simulink model "fusionAlg"  (R2018b)
settings: Solver=FixedStepDiscrete  StartTime=0.0  StopTime=inf  FixedStep=0.01  RelTol=1e-3
PostLoadFcn:
  | if any(exist('dsrtsu_mdlpostloadfcn', 'file') ~= 0), dsrtsu_mdlpostloadfcn('Execute', bdroot); end
model workspace (MAT data in the model file):
  handle : class17 (value not decoded)
(part 8 of 24)

== system fusionAlg/FUSION /FUS_DataAdapter/VisionAdapter/ObjAdapter/Obj_39 ==
  EyeQ4_Obj_01 : Inport
  Bus Creator1 : BusCreator  Inputs=21  OutDataTypeStr=Bus: FUS_VISION_OBJ_ST
      settings: InheritFromInputs=off
  Bus Selector : BusSelector  OutputSignals=OBJ_ID,OBJ_Measuring_Status,OBJ_Object_Age,OBJ_Object_Class,OBJ_Class_Probability,OBJ_Lat_Distance,OBJ_Lat_Distance_STD,OBJ_Long_Distance,OBJ_Long_Distance_STD,OBJ_Abs_Long_Velocity,OBJ_Abs_Long_Velocity_STD,OBJ_Abs_Lat_Velocity,OBJ_Abs_Lat_Velocity_STD,OBJ_Angle_Mid,OBJ_Angle_Mid_STD,OBJ_Inv_TTC,OBJ_Inv_TTC_STD,OBJ_Abs_Long_Acc,OBJ_Abs_Long_Acc_STD,OBJ_Abs_Lat_Acc,OBJ_Abs_Lat_Acc_STD,OBJ_Length,OBJ_Width,OBJ_Height,OBJ_Heading
  Constant : Constant  OutDataTypeStr=single
  Constant1 : Constant  Value=0  OutDataTypeStr=uint8
  Constant2 : Constant  OutDataTypeStr=single
  Constant3 : Constant  Value=0  OutDataTypeStr=single
  Constant4 : Constant  Value=0  OutDataTypeStr=single
  Data Type Conversion : DataTypeConversion  OutDataTypeStr=uint32
  Data Type Conversion3 : DataTypeConversion  OutDataTypeStr=uint32
  Obj_01_Agge : Subsystem
  Obj_01_boundarhy : Subsystem
  Subsystem : Subsystem
  Subsystem1 : Subsystem
  Subsystem2 : Subsystem
  Subsystem3 : Subsystem
  Subsystem4 : Subsystem
  Subsystem5 : Subsystem
  Subsystem6 : Subsystem
  Subsystem7 : Subsystem
  Subsystem8 : Subsystem
  Obj_01_st : Outport  OutDataTypeStr=Bus: FUS_VISION_OBJ_ST
  wires:
  Bus Selector/1 -> Data Type Conversion/1  "<OBJ_ID>"
  Bus Selector/3 -> Obj_01_Agge/1(<OBJ_Object_Age>)  "<OBJ_Object_Age>"
  Obj_01_Agge/1(Obj_01_Age) -> Bus Creator1/3  "Obj_Age"
  Obj_01_boundarhy/1(Obj_01_boundary) -> Bus Creator1/4  "Obj_Boundary"
  Bus Selector/5 -> Data Type Conversion3/1  "<OBJ_Class_Probability>"
  Bus Selector/6 -> Subsystem/1(<OBJ_Lat_Distance>)  "<OBJ_Lat_Distance>"
  Bus Selector/7 -> Subsystem/2(<OBJ_Lat_Distance_STD>)  "<OBJ_Lat_Distance_STD>"
  Bus Selector/8 -> Subsystem/3(<OBJ_Long_Distance>)  "<OBJ_Long_Distance>"
  Bus Selector/9 -> Subsystem/4(<OBJ_Long_Distance_STD>)  "<OBJ_Long_Distance_STD>"
  Subsystem/1(Obj_01_coordinate) -> Bus Creator1/7  "Obj_Coor"
  Bus Selector/10 -> Subsystem1/1(<OBJ_Abs_Long_Velocity>)  "<OBJ_Abs_Long_Velocity>"
  Bus Selector/11 -> Subsystem1/2(<OBJ_Abs_Long_Velocity_STD>)  "<OBJ_Abs_Long_Velocity_STD>"
  Bus Selector/12 -> Subsystem1/3(<OBJ_Abs_Lat_Velocity>)  "<OBJ_Abs_Lat_Velocity>"
  Bus Selector/13 -> Subsystem1/4(<OBJ_Abs_Lat_Velocity_STD>)  "<OBJ_Abs_Lat_Velocity_STD>"
  Subsystem1/1(Out1) -> Bus Creator1/8  "Obj_Vel"
  Bus Selector/14 -> Subsystem2/1(<OBJ_Angle_Mid>)  "<OBJ_Angle_Mid>"
  Bus Selector/15 -> Subsystem2/2(<OBJ_Angle_Mid_STD>)  "<OBJ_Angle_Mid_STD>"
  Subsystem2/1(Out1) -> Bus Creator1/9  "Obj_Anage"
  Bus Selector/16 -> Bus Creator1/10  "<OBJ_Inv_TTC>"
  Bus Selector/17 -> Bus Creator1/11  "<OBJ_Inv_TTC_STD>"
  Bus Selector/18 -> Subsystem3/1(<OBJ_Abs_Long_Acc>)  "<OBJ_Abs_Long_Acc>"
  Bus Selector/19 -> Subsystem3/2(<OBJ_Abs_Long_Acc_STD>)  "<OBJ_Abs_Long_Acc_STD>"
  Bus Selector/20 -> Subsystem3/3(<OBJ_Abs_Lat_Acc>)  "<OBJ_Abs_Lat_Acc>"
  Bus Selector/21 -> Subsystem3/4(<OBJ_Abs_Lat_Acc_STD>)  "<OBJ_Abs_Lat_Acc_STD>"
  Subsystem3/1(Out1) -> Bus Creator1/12  "Obj_Acc"
  Constant/1 -> Bus Creator1/13  "existProb"
  Bus Selector/22 -> Subsystem4/1(<OBJ_Length>)  "<OBJ_Length>"
  Bus Selector/23 -> Subsystem4/2(<OBJ_Width>)  "<OBJ_Width>"
  Bus Selector/24 -> Subsystem4/3(<OBJ_Height>)  "<OBJ_Height>"
  Subsystem4/1(Out1) -> Bus Creator1/14  "Obj_BoxSize"
  Constant1/1 -> Bus Creator1/15  "AngelOfObj"
  Subsystem5/1(reserved1) -> Bus Creator1/16
  Bus Selector/25 -> Bus Creator1/17  "<OBJ_Heading>"
  Constant2/1 -> Bus Creator1/18
  Constant3/1 -> Bus Creator1/19
  Constant4/1 -> Bus Creator1/20
  Subsystem6/1(reserved2) -> Bus Creator1/21
  EyeQ4_Obj_01/1 -> Bus Selector/1
  Bus Creator1/1 -> Obj_01_st/1
  Data Type Conversion/1 -> Bus Creator1/1
  Data Type Conversion3/1 -> Bus Creator1/6  "Obj_TypeConf"
  Bus Selector/2 -> Subsystem7/1(<OBJ_Measuring_Status>)  "<OBJ_Measuring_Status>"
  Subsystem7/1(Obj_Status) -> Bus Creator1/2  "Obj_Status"
  Bus Selector/4 -> Subsystem8/1(<OBJ_Object_Class>)  "<OBJ_Object_Class>"
  Subsystem8/1(Obj_Type) -> Bus Creator1/5  "Obj_Type"

== system fusionAlg/FUSION /FUS_DataAdapter/VisionAdapter/ObjAdapter/Obj_4 ==
  EyeQ4_Obj_01 : Inport
  Bus Creator1 : BusCreator  Inputs=21  OutDataTypeStr=Bus: FUS_VISION_OBJ_ST
      settings: InheritFromInputs=off
  Bus Selector : BusSelector  OutputSignals=OBJ_ID,OBJ_Measuring_Status,OBJ_Object_Age,OBJ_Object_Class,OBJ_Class_Probability,OBJ_Lat_Distance,OBJ_Lat_Distance_STD,OBJ_Long_Distance,OBJ_Long_Distance_STD,OBJ_Abs_Long_Velocity,OBJ_Abs_Long_Velocity_STD,OBJ_Abs_Lat_Velocity,OBJ_Abs_Lat_Velocity_STD,OBJ_Angle_Mid,OBJ_Angle_Mid_STD,OBJ_Inv_TTC,OBJ_Inv_TTC_STD,OBJ_Abs_Long_Acc,OBJ_Abs_Long_Acc_STD,OBJ_Abs_Lat_Acc,OBJ_Abs_Lat_Acc_STD,OBJ_Length,OBJ_Width,OBJ_Height,OBJ_Heading
  Constant : Constant  OutDataTypeStr=single
  Constant1 : Constant  Value=0  OutDataTypeStr=uint8
  Constant2 : Constant  OutDataTypeStr=single
  Constant3 : Constant  Value=0  OutDataTypeStr=single
  Constant4 : Constant  Value=0  OutDataTypeStr=single
  Data Type Conversion : DataTypeConversion  OutDataTypeStr=uint32
  Data Type Conversion3 : DataTypeConversion  OutDataTypeStr=uint32
  Obj_01_Agge : Subsystem
  Obj_01_boundarhy : Subsystem
  Subsystem : Subsystem
  Subsystem1 : Subsystem
  Subsystem2 : Subsystem
  Subsystem3 : Subsystem
  Subsystem4 : Subsystem
  Subsystem5 : Subsystem
  Subsystem6 : Subsystem
  Subsystem7 : Subsystem
  Subsystem8 : Subsystem
  Obj_01_st : Outport  OutDataTypeStr=Bus: FUS_VISION_OBJ_ST
  wires:
  Bus Selector/1 -> Data Type Conversion/1  "<OBJ_ID>"
  Bus Selector/3 -> Obj_01_Agge/1(<OBJ_Object_Age>)  "<OBJ_Object_Age>"
  Obj_01_Agge/1(Obj_01_Age) -> Bus Creator1/3  "Obj_Age"
  Obj_01_boundarhy/1(Obj_01_boundary) -> Bus Creator1/4  "Obj_Boundary"
  Bus Selector/5 -> Data Type Conversion3/1  "<OBJ_Class_Probability>"
  Bus Selector/6 -> Subsystem/1(<OBJ_Lat_Distance>)  "<OBJ_Lat_Distance>"
  Bus Selector/7 -> Subsystem/2(<OBJ_Lat_Distance_STD>)  "<OBJ_Lat_Distance_STD>"
  Bus Selector/8 -> Subsystem/3(<OBJ_Long_Distance>)  "<OBJ_Long_Distance>"
  Bus Selector/9 -> Subsystem/4(<OBJ_Long_Distance_STD>)  "<OBJ_Long_Distance_STD>"
  Subsystem/1(Obj_01_coordinate) -> Bus Creator1/7  "Obj_Coor"
  Bus Selector/10 -> Subsystem1/1(<OBJ_Abs_Long_Velocity>)  "<OBJ_Abs_Long_Velocity>"
  Bus Selector/11 -> Subsystem1/2(<OBJ_Abs_Long_Velocity_STD>)  "<OBJ_Abs_Long_Velocity_STD>"
  Bus Selector/12 -> Subsystem1/3(<OBJ_Abs_Lat_Velocity>)  "<OBJ_Abs_Lat_Velocity>"
  Bus Selector/13 -> Subsystem1/4(<OBJ_Abs_Lat_Velocity_STD>)  "<OBJ_Abs_Lat_Velocity_STD>"
  Subsystem1/1(Out1) -> Bus Creator1/8  "Obj_Vel"
  Bus Selector/14 -> Subsystem2/1(<OBJ_Angle_Mid>)  "<OBJ_Angle_Mid>"
  Bus Selector/15 -> Subsystem2/2(<OBJ_Angle_Mid_STD>)  "<OBJ_Angle_Mid_STD>"
  Subsystem2/1(Out1) -> Bus Creator1/9  "Obj_Anage"
  Bus Selector/16 -> Bus Creator1/10  "<OBJ_Inv_TTC>"
  Bus Selector/17 -> Bus Creator1/11  "<OBJ_Inv_TTC_STD>"
  Bus Selector/18 -> Subsystem3/1(<OBJ_Abs_Long_Acc>)  "<OBJ_Abs_Long_Acc>"
  Bus Selector/19 -> Subsystem3/2(<OBJ_Abs_Long_Acc_STD>)  "<OBJ_Abs_Long_Acc_STD>"
  Bus Selector/20 -> Subsystem3/3(<OBJ_Abs_Lat_Acc>)  "<OBJ_Abs_Lat_Acc>"
  Bus Selector/21 -> Subsystem3/4(<OBJ_Abs_Lat_Acc_STD>)  "<OBJ_Abs_Lat_Acc_STD>"
  Subsystem3/1(Out1) -> Bus Creator1/12  "Obj_Acc"
  Constant/1 -> Bus Creator1/13  "existProb"
  Bus Selector/22 -> Subsystem4/1(<OBJ_Length>)  "<OBJ_Length>"
  Bus Selector/23 -> Subsystem4/2(<OBJ_Width>)  "<OBJ_Width>"
  Bus Selector/24 -> Subsystem4/3(<OBJ_Height>)  "<OBJ_Height>"
  Subsystem4/1(Out1) -> Bus Creator1/14  "Obj_BoxSize"
  Constant1/1 -> Bus Creator1/15  "AngelOfObj"
  Subsystem5/1(reserved1) -> Bus Creator1/16
  Bus Selector/25 -> Bus Creator1/17  "<OBJ_Heading>"
  Constant2/1 -> Bus Creator1/18
  Constant3/1 -> Bus Creator1/19
  Constant4/1 -> Bus Creator1/20
  Subsystem6/1(reserved2) -> Bus Creator1/21
  EyeQ4_Obj_01/1 -> Bus Selector/1
  Bus Creator1/1 -> Obj_01_st/1
  Data Type Conversion/1 -> Bus Creator1/1
  Data Type Conversion3/1 -> Bus Creator1/6  "Obj_TypeConf"
  Bus Selector/2 -> Subsystem7/1(<OBJ_Measuring_Status>)  "<OBJ_Measuring_Status>"
  Subsystem7/1(Obj_Status) -> Bus Creator1/2  "Obj_Status"
  Bus Selector/4 -> Subsystem8/1(<OBJ_Object_Class>)  "<OBJ_Object_Class>"
  Subsystem8/1(Obj_Type) -> Bus Creator1/5  "Obj_Type"

== system fusionAlg/FUSION /FUS_DataAdapter/VisionAdapter/ObjAdapter/Obj_40 ==
  EyeQ4_Obj_01 : Inport
  Bus Creator1 : BusCreator  Inputs=21  OutDataTypeStr=Bus: FUS_VISION_OBJ_ST
      settings: InheritFromInputs=off
  Bus Selector : BusSelector  OutputSignals=OBJ_ID,OBJ_Measuring_Status,OBJ_Object_Age,OBJ_Object_Class,OBJ_Class_Probability,OBJ_Lat_Distance,OBJ_Lat_Distance_STD,OBJ_Long_Distance,OBJ_Long_Distance_STD,OBJ_Abs_Long_Velocity,OBJ_Abs_Long_Velocity_STD,OBJ_Abs_Lat_Velocity,OBJ_Abs_Lat_Velocity_STD,OBJ_Angle_Mid,OBJ_Angle_Mid_STD,OBJ_Inv_TTC,OBJ_Inv_TTC_STD,OBJ_Abs_Long_Acc,OBJ_Abs_Long_Acc_STD,OBJ_Abs_Lat_Acc,OBJ_Abs_Lat_Acc_STD,OBJ_Length,OBJ_Width,OBJ_Height,OBJ_Heading
  Constant : Constant  OutDataTypeStr=single
  Constant1 : Constant  Value=0  OutDataTypeStr=uint8
  Constant2 : Constant  OutDataTypeStr=single
  Constant3 : Constant  Value=0  OutDataTypeStr=single
  Constant4 : Constant  Value=0  OutDataTypeStr=single
  Data Type Conversion : DataTypeConversion  OutDataTypeStr=uint32
  Data Type Conversion3 : DataTypeConversion  OutDataTypeStr=uint32
  Obj_01_Agge : Subsystem
  Obj_01_boundarhy : Subsystem
  Subsystem : Subsystem
  Subsystem1 : Subsystem
  Subsystem2 : Subsystem
  Subsystem3 : Subsystem
  Subsystem4 : Subsystem
  Subsystem5 : Subsystem
  Subsystem6 : Subsystem
  Subsystem7 : Subsystem
  Subsystem8 : Subsystem
  Obj_01_st : Outport  OutDataTypeStr=Bus: FUS_VISION_OBJ_ST
  wires:
  Bus Selector/1 -> Data Type Conversion/1  "<OBJ_ID>"
  Bus Selector/3 -> Obj_01_Agge/1(<OBJ_Object_Age>)  "<OBJ_Object_Age>"
  Obj_01_Agge/1(Obj_01_Age) -> Bus Creator1/3  "Obj_Age"
  Obj_01_boundarhy/1(Obj_01_boundary) -> Bus Creator1/4  "Obj_Boundary"
  Bus Selector/5 -> Data Type Conversion3/1  "<OBJ_Class_Probability>"
  Bus Selector/6 -> Subsystem/1(<OBJ_Lat_Distance>)  "<OBJ_Lat_Distance>"
  Bus Selector/7 -> Subsystem/2(<OBJ_Lat_Distance_STD>)  "<OBJ_Lat_Distance_STD>"
  Bus Selector/8 -> Subsystem/3(<OBJ_Long_Distance>)  "<OBJ_Long_Distance>"
  Bus Selector/9 -> Subsystem/4(<OBJ_Long_Distance_STD>)  "<OBJ_Long_Distance_STD>"
  Subsystem/1(Obj_01_coordinate) -> Bus Creator1/7  "Obj_Coor"
  Bus Selector/10 -> Subsystem1/1(<OBJ_Abs_Long_Velocity>)  "<OBJ_Abs_Long_Velocity>"
  Bus Selector/11 -> Subsystem1/2(<OBJ_Abs_Long_Velocity_STD>)  "<OBJ_Abs_Long_Velocity_STD>"
  Bus Selector/12 -> Subsystem1/3(<OBJ_Abs_Lat_Velocity>)  "<OBJ_Abs_Lat_Velocity>"
  Bus Selector/13 -> Subsystem1/4(<OBJ_Abs_Lat_Velocity_STD>)  "<OBJ_Abs_Lat_Velocity_STD>"
  Subsystem1/1(Out1) -> Bus Creator1/8  "Obj_Vel"
  Bus Selector/14 -> Subsystem2/1(<OBJ_Angle_Mid>)  "<OBJ_Angle_Mid>"
  Bus Selector/15 -> Subsystem2/2(<OBJ_Angle_Mid_STD>)  "<OBJ_Angle_Mid_STD>"
  Subsystem2/1(Out1) -> Bus Creator1/9  "Obj_Anage"
  Bus Selector/16 -> Bus Creator1/10  "<OBJ_Inv_TTC>"
  Bus Selector/17 -> Bus Creator1/11  "<OBJ_Inv_TTC_STD>"
  Bus Selector/18 -> Subsystem3/1(<OBJ_Abs_Long_Acc>)  "<OBJ_Abs_Long_Acc>"
  Bus Selector/19 -> Subsystem3/2(<OBJ_Abs_Long_Acc_STD>)  "<OBJ_Abs_Long_Acc_STD>"
  Bus Selector/20 -> Subsystem3/3(<OBJ_Abs_Lat_Acc>)  "<OBJ_Abs_Lat_Acc>"
  Bus Selector/21 -> Subsystem3/4(<OBJ_Abs_Lat_Acc_STD>)  "<OBJ_Abs_Lat_Acc_STD>"
  Subsystem3/1(Out1) -> Bus Creator1/12  "Obj_Acc"
  Constant/1 -> Bus Creator1/13  "existProb"
  Bus Selector/22 -> Subsystem4/1(<OBJ_Length>)  "<OBJ_Length>"
  Bus Selector/23 -> Subsystem4/2(<OBJ_Width>)  "<OBJ_Width>"
  Bus Selector/24 -> Subsystem4/3(<OBJ_Height>)  "<OBJ_Height>"
  Subsystem4/1(Out1) -> Bus Creator1/14  "Obj_BoxSize"
  Constant1/1 -> Bus Creator1/15  "AngelOfObj"
  Subsystem5/1(reserved1) -> Bus Creator1/16
  Bus Selector/25 -> Bus Creator1/17  "<OBJ_Heading>"
  Constant2/1 -> Bus Creator1/18
  Constant3/1 -> Bus Creator1/19
  Constant4/1 -> Bus Creator1/20
  Subsystem6/1(reserved2) -> Bus Creator1/21
  EyeQ4_Obj_01/1 -> Bus Selector/1
  Bus Creator1/1 -> Obj_01_st/1
  Data Type Conversion/1 -> Bus Creator1/1
  Data Type Conversion3/1 -> Bus Creator1/6  "Obj_TypeConf"
  Bus Selector/2 -> Subsystem7/1(<OBJ_Measuring_Status>)  "<OBJ_Measuring_Status>"
  Subsystem7/1(Obj_Status) -> Bus Creator1/2  "Obj_Status"
  Bus Selector/4 -> Subsystem8/1(<OBJ_Object_Class>)  "<OBJ_Object_Class>"
  Subsystem8/1(Obj_Type) -> Bus Creator1/5  "Obj_Type"

== system fusionAlg/FUSION /FUS_DataAdapter/VisionAdapter/ObjAdapter/Obj_5 ==
  EyeQ4_Obj_01 : Inport
  Bus Creator1 : BusCreator  Inputs=21  OutDataTypeStr=Bus: FUS_VISION_OBJ_ST
      settings: InheritFromInputs=off
  Bus Selector : BusSelector  OutputSignals=OBJ_ID,OBJ_Measuring_Status,OBJ_Object_Age,OBJ_Object_Class,OBJ_Class_Probability,OBJ_Lat_Distance,OBJ_Lat_Distance_STD,OBJ_Long_Distance,OBJ_Long_Distance_STD,OBJ_Abs_Long_Velocity,OBJ_Abs_Long_Velocity_STD,OBJ_Abs_Lat_Velocity,OBJ_Abs_Lat_Velocity_STD,OBJ_Angle_Mid,OBJ_Angle_Mid_STD,OBJ_Inv_TTC,OBJ_Inv_TTC_STD,OBJ_Abs_Long_Acc,OBJ_Abs_Long_Acc_STD,OBJ_Abs_Lat_Acc,OBJ_Abs_Lat_Acc_STD,OBJ_Length,OBJ_Width,OBJ_Height,OBJ_Heading
  Constant : Constant  OutDataTypeStr=single
  Constant1 : Constant  Value=0  OutDataTypeStr=uint8
  Constant2 : Constant  OutDataTypeStr=single
  Constant3 : Constant  Value=0  OutDataTypeStr=single
  Constant4 : Constant  Value=0  OutDataTypeStr=single
  Data Type Conversion : DataTypeConversion  OutDataTypeStr=uint32
  Data Type Conversion3 : DataTypeConversion  OutDataTypeStr=uint32
  Obj_01_Agge : Subsystem
  Obj_01_boundarhy : Subsystem
  Subsystem : Subsystem
  Subsystem1 : Subsystem
  Subsystem2 : Subsystem
  Subsystem3 : Subsystem
  Subsystem4 : Subsystem
  Subsystem5 : Subsystem
  Subsystem6 : Subsystem
  Subsystem7 : Subsystem
  Subsystem8 : Subsystem
  Obj_01_st : Outport  OutDataTypeStr=Bus: FUS_VISION_OBJ_ST
  wires:
  Bus Selector/1 -> Data Type Conversion/1  "<OBJ_ID>"
  Bus Selector/3 -> Obj_01_Agge/1(<OBJ_Object_Age>)  "<OBJ_Object_Age>"
  Obj_01_Agge/1(Obj_01_Age) -> Bus Creator1/3  "Obj_Age"
  Obj_01_boundarhy/1(Obj_01_boundary) -> Bus Creator1/4  "Obj_Boundary"
  Bus Selector/5 -> Data Type Conversion3/1  "<OBJ_Class_Probability>"
  Bus Selector/6 -> Subsystem/1(<OBJ_Lat_Distance>)  "<OBJ_Lat_Distance>"
  Bus Selector/7 -> Subsystem/2(<OBJ_Lat_Distance_STD>)  "<OBJ_Lat_Distance_STD>"
  Bus Selector/8 -> Subsystem/3(<OBJ_Long_Distance>)  "<OBJ_Long_Distance>"
  Bus Selector/9 -> Subsystem/4(<OBJ_Long_Distance_STD>)  "<OBJ_Long_Distance_STD>"
  Subsystem/1(Obj_01_coordinate) -> Bus Creator1/7  "Obj_Coor"
  Bus Selector/10 -> Subsystem1/1(<OBJ_Abs_Long_Velocity>)  "<OBJ_Abs_Long_Velocity>"
  Bus Selector/11 -> Subsystem1/2(<OBJ_Abs_Long_Velocity_STD>)  "<OBJ_Abs_Long_Velocity_STD>"
  Bus Selector/12 -> Subsystem1/3(<OBJ_Abs_Lat_Velocity>)  "<OBJ_Abs_Lat_Velocity>"
  Bus Selector/13 -> Subsystem1/4(<OBJ_Abs_Lat_Velocity_STD>)  "<OBJ_Abs_Lat_Velocity_STD>"
  Subsystem1/1(Out1) -> Bus Creator1/8  "Obj_Vel"
  Bus Selector/14 -> Subsystem2/1(<OBJ_Angle_Mid>)  "<OBJ_Angle_Mid>"
  Bus Selector/15 -> Subsystem2/2(<OBJ_Angle_Mid_STD>)  "<OBJ_Angle_Mid_STD>"
  Subsystem2/1(Out1) -> Bus Creator1/9  "Obj_Anage"
  Bus Selector/16 -> Bus Creator1/10  "<OBJ_Inv_TTC>"
  Bus Selector/17 -> Bus Creator1/11  "<OBJ_Inv_TTC_STD>"
  Bus Selector/18 -> Subsystem3/1(<OBJ_Abs_Long_Acc>)  "<OBJ_Abs_Long_Acc>"
  Bus Selector/19 -> Subsystem3/2(<OBJ_Abs_Long_Acc_STD>)  "<OBJ_Abs_Long_Acc_STD>"
  Bus Selector/20 -> Subsystem3/3(<OBJ_Abs_Lat_Acc>)  "<OBJ_Abs_Lat_Acc>"
  Bus Selector/21 -> Subsystem3/4(<OBJ_Abs_Lat_Acc_STD>)  "<OBJ_Abs_Lat_Acc_STD>"
  Subsystem3/1(Out1) -> Bus Creator1/12  "Obj_Acc"
  Constant/1 -> Bus Creator1/13  "existProb"
  Bus Selector/22 -> Subsystem4/1(<OBJ_Length>)  "<OBJ_Length>"
  Bus Selector/23 -> Subsystem4/2(<OBJ_Width>)  "<OBJ_Width>"
  Bus Selector/24 -> Subsystem4/3(<OBJ_Height>)  "<OBJ_Height>"
  Subsystem4/1(Out1) -> Bus Creator1/14  "Obj_BoxSize"
  Constant1/1 -> Bus Creator1/15  "AngelOfObj"
  Subsystem5/1(reserved1) -> Bus Creator1/16
  Bus Selector/25 -> Bus Creator1/17  "<OBJ_Heading>"
  Constant2/1 -> Bus Creator1/18
  Constant3/1 -> Bus Creator1/19
  Constant4/1 -> Bus Creator1/20
  Subsystem6/1(reserved2) -> Bus Creator1/21
  EyeQ4_Obj_01/1 -> Bus Selector/1
  Bus Creator1/1 -> Obj_01_st/1
  Data Type Conversion/1 -> Bus Creator1/1
  Data Type Conversion3/1 -> Bus Creator1/6  "Obj_TypeConf"
  Bus Selector/2 -> Subsystem7/1(<OBJ_Measuring_Status>)  "<OBJ_Measuring_Status>"
  Subsystem7/1(Obj_Status) -> Bus Creator1/2  "Obj_Status"
  Bus Selector/4 -> Subsystem8/1(<OBJ_Object_Class>)  "<OBJ_Object_Class>"
  Subsystem8/1(Obj_Type) -> Bus Creator1/5  "Obj_Type"

== system fusionAlg/FUSION /FUS_DataAdapter/VisionAdapter/ObjAdapter/Obj_6 ==
  EyeQ4_Obj_01 : Inport
  Bus Creator1 : BusCreator  Inputs=21  OutDataTypeStr=Bus: FUS_VISION_OBJ_ST
      settings: InheritFromInputs=off
  Bus Selector : BusSelector  OutputSignals=OBJ_ID,OBJ_Measuring_Status,OBJ_Object_Age,OBJ_Object_Class,OBJ_Class_Probability,OBJ_Lat_Distance,OBJ_Lat_Distance_STD,OBJ_Long_Distance,OBJ_Long_Distance_STD,OBJ_Abs_Long_Velocity,OBJ_Abs_Long_Velocity_STD,OBJ_Abs_Lat_Velocity,OBJ_Abs_Lat_Velocity_STD,OBJ_Angle_Mid,OBJ_Angle_Mid_STD,OBJ_Inv_TTC,OBJ_Inv_TTC_STD,OBJ_Abs_Long_Acc,OBJ_Abs_Long_Acc_STD,OBJ_Abs_Lat_Acc,OBJ_Abs_Lat_Acc_STD,OBJ_Length,OBJ_Width,OBJ_Height,OBJ_Heading
  Constant : Constant  OutDataTypeStr=single
  Constant1 : Constant  Value=0  OutDataTypeStr=uint8
  Constant2 : Constant  OutDataTypeStr=single
  Constant3 : Constant  Value=0  OutDataTypeStr=single
  Constant4 : Constant  Value=0  OutDataTypeStr=single
  Data Type Conversion : DataTypeConversion  OutDataTypeStr=uint32
  Data Type Conversion3 : DataTypeConversion  OutDataTypeStr=uint32
  Obj_01_Agge : Subsystem
  Obj_01_boundarhy : Subsystem
  Subsystem : Subsystem
  Subsystem1 : Subsystem
  Subsystem2 : Subsystem
  Subsystem3 : Subsystem
  Subsystem4 : Subsystem
  Subsystem5 : Subsystem
  Subsystem6 : Subsystem
  Subsystem7 : Subsystem
  Subsystem8 : Subsystem
  Obj_01_st : Outport  OutDataTypeStr=Bus: FUS_VISION_OBJ_ST
  wires:
  Bus Selector/1 -> Data Type Conversion/1  "<OBJ_ID>"
  Bus Selector/3 -> Obj_01_Agge/1(<OBJ_Object_Age>)  "<OBJ_Object_Age>"
  Obj_01_Agge/1(Obj_01_Age) -> Bus Creator1/3  "Obj_Age"
  Obj_01_boundarhy/1(Obj_01_boundary) -> Bus Creator1/4  "Obj_Boundary"
  Bus Selector/5 -> Data Type Conversion3/1  "<OBJ_Class_Probability>"
  Bus Selector/6 -> Subsystem/1(<OBJ_Lat_Distance>)  "<OBJ_Lat_Distance>"
  Bus Selector/7 -> Subsystem/2(<OBJ_Lat_Distance_STD>)  "<OBJ_Lat_Distance_STD>"
  Bus Selector/8 -> Subsystem/3(<OBJ_Long_Distance>)  "<OBJ_Long_Distance>"
  Bus Selector/9 -> Subsystem/4(<OBJ_Long_Distance_STD>)  "<OBJ_Long_Distance_STD>"
  Subsystem/1(Obj_01_coordinate) -> Bus Creator1/7  "Obj_Coor"
  Bus Selector/10 -> Subsystem1/1(<OBJ_Abs_Long_Velocity>)  "<OBJ_Abs_Long_Velocity>"
  Bus Selector/11 -> Subsystem1/2(<OBJ_Abs_Long_Velocity_STD>)  "<OBJ_Abs_Long_Velocity_STD>"
  Bus Selector/12 -> Subsystem1/3(<OBJ_Abs_Lat_Velocity>)  "<OBJ_Abs_Lat_Velocity>"
  Bus Selector/13 -> Subsystem1/4(<OBJ_Abs_Lat_Velocity_STD>)  "<OBJ_Abs_Lat_Velocity_STD>"
  Subsystem1/1(Out1) -> Bus Creator1/8  "Obj_Vel"
  Bus Selector/14 -> Subsystem2/1(<OBJ_Angle_Mid>)  "<OBJ_Angle_Mid>"
  Bus Selector/15 -> Subsystem2/2(<OBJ_Angle_Mid_STD>)  "<OBJ_Angle_Mid_STD>"
  Subsystem2/1(Out1) -> Bus Creator1/9  "Obj_Anage"
  Bus Selector/16 -> Bus Creator1/10  "<OBJ_Inv_TTC>"
  Bus Selector/17 -> Bus Creator1/11  "<OBJ_Inv_TTC_STD>"
  Bus Selector/18 -> Subsystem3/1(<OBJ_Abs_Long_Acc>)  "<OBJ_Abs_Long_Acc>"
  Bus Selector/19 -> Subsystem3/2(<OBJ_Abs_Long_Acc_STD>)  "<OBJ_Abs_Long_Acc_STD>"
  Bus Selector/20 -> Subsystem3/3(<OBJ_Abs_Lat_Acc>)  "<OBJ_Abs_Lat_Acc>"
  Bus Selector/21 -> Subsystem3/4(<OBJ_Abs_Lat_Acc_STD>)  "<OBJ_Abs_Lat_Acc_STD>"
  Subsystem3/1(Out1) -> Bus Creator1/12  "Obj_Acc"
  Constant/1 -> Bus Creator1/13  "existProb"
  Bus Selector/22 -> Subsystem4/1(<OBJ_Length>)  "<OBJ_Length>"
  Bus Selector/23 -> Subsystem4/2(<OBJ_Width>)  "<OBJ_Width>"
  Bus Selector/24 -> Subsystem4/3(<OBJ_Height>)  "<OBJ_Height>"
  Subsystem4/1(Out1) -> Bus Creator1/14  "Obj_BoxSize"
  Constant1/1 -> Bus Creator1/15  "AngelOfObj"
  Subsystem5/1(reserved1) -> Bus Creator1/16
  Bus Selector/25 -> Bus Creator1/17  "<OBJ_Heading>"
  Constant2/1 -> Bus Creator1/18
  Constant3/1 -> Bus Creator1/19
  Constant4/1 -> Bus Creator1/20
  Subsystem6/1(reserved2) -> Bus Creator1/21
  EyeQ4_Obj_01/1 -> Bus Selector/1
  Bus Creator1/1 -> Obj_01_st/1
  Data Type Conversion/1 -> Bus Creator1/1
  Data Type Conversion3/1 -> Bus Creator1/6  "Obj_TypeConf"
  Bus Selector/2 -> Subsystem7/1(<OBJ_Measuring_Status>)  "<OBJ_Measuring_Status>"
  Subsystem7/1(Obj_Status) -> Bus Creator1/2  "Obj_Status"
  Bus Selector/4 -> Subsystem8/1(<OBJ_Object_Class>)  "<OBJ_Object_Class>"
  Subsystem8/1(Obj_Type) -> Bus Creator1/5  "Obj_Type"

== system fusionAlg/FUSION /FUS_DataAdapter/VisionAdapter/ObjAdapter/Obj_7 ==
  EyeQ4_Obj_01 : Inport
  Bus Creator1 : BusCreator  Inputs=21  OutDataTypeStr=Bus: FUS_VISION_OBJ_ST
      settings: InheritFromInputs=off
  Bus Selector : BusSelector  OutputSignals=OBJ_ID,OBJ_Measuring_Status,OBJ_Object_Age,OBJ_Object_Class,OBJ_Class_Probability,OBJ_Lat_Distance,OBJ_Lat_Distance_STD,OBJ_Long_Distance,OBJ_Long_Distance_STD,OBJ_Abs_Long_Velocity,OBJ_Abs_Long_Velocity_STD,OBJ_Abs_Lat_Velocity,OBJ_Abs_Lat_Velocity_STD,OBJ_Angle_Mid,OBJ_Angle_Mid_STD,OBJ_Inv_TTC,OBJ_Inv_TTC_STD,OBJ_Abs_Long_Acc,OBJ_Abs_Long_Acc_STD,OBJ_Abs_Lat_Acc,OBJ_Abs_Lat_Acc_STD,OBJ_Length,OBJ_Width,OBJ_Height,OBJ_Heading
  Constant : Constant  OutDataTypeStr=single
  Constant1 : Constant  Value=0  OutDataTypeStr=uint8
  Constant2 : Constant  OutDataTypeStr=single
  Constant3 : Constant  Value=0  OutDataTypeStr=single
  Constant4 : Constant  Value=0  OutDataTypeStr=single
  Data Type Conversion : DataTypeConversion  OutDataTypeStr=uint32
  Data Type Conversion3 : DataTypeConversion  OutDataTypeStr=uint32
  Obj_01_Agge : Subsystem
  Obj_01_boundarhy : Subsystem
  Subsystem : Subsystem
  Subsystem1 : Subsystem
  Subsystem2 : Subsystem
  Subsystem3 : Subsystem
  Subsystem4 : Subsystem
  Subsystem5 : Subsystem
  Subsystem6 : Subsystem
  Subsystem7 : Subsystem
  Subsystem8 : Subsystem
  Obj_01_st : Outport  OutDataTypeStr=Bus: FUS_VISION_OBJ_ST
  wires:
  Bus Selector/1 -> Data Type Conversion/1  "<OBJ_ID>"
  Bus Selector/3 -> Obj_01_Agge/1(<OBJ_Object_Age>)  "<OBJ_Object_Age>"
  Obj_01_Agge/1(Obj_01_Age) -> Bus Creator1/3  "Obj_Age"
  Obj_01_boundarhy/1(Obj_01_boundary) -> Bus Creator1/4  "Obj_Boundary"
  Bus Selector/5 -> Data Type Conversion3/1  "<OBJ_Class_Probability>"
  Bus Selector/6 -> Subsystem/1(<OBJ_Lat_Distance>)  "<OBJ_Lat_Distance>"
  Bus Selector/7 -> Subsystem/2(<OBJ_Lat_Distance_STD>)  "<OBJ_Lat_Distance_STD>"
  Bus Selector/8 -> Subsystem/3(<OBJ_Long_Distance>)  "<OBJ_Long_Distance>"
  Bus Selector/9 -> Subsystem/4(<OBJ_Long_Distance_STD>)  "<OBJ_Long_Distance_STD>"
  Subsystem/1(Obj_01_coordinate) -> Bus Creator1/7  "Obj_Coor"
  Bus Selector/10 -> Subsystem1/1(<OBJ_Abs_Long_Velocity>)  "<OBJ_Abs_Long_Velocity>"
  Bus Selector/11 -> Subsystem1/2(<OBJ_Abs_Long_Velocity_STD>)  "<OBJ_Abs_Long_Velocity_STD>"
  Bus Selector/12 -> Subsystem1/3(<OBJ_Abs_Lat_Velocity>)  "<OBJ_Abs_Lat_Velocity>"
  Bus Selector/13 -> Subsystem1/4(<OBJ_Abs_Lat_Velocity_STD>)  "<OBJ_Abs_Lat_Velocity_STD>"
  Subsystem1/1(Out1) -> Bus Creator1/8  "Obj_Vel"
  Bus Selector/14 -> Subsystem2/1(<OBJ_Angle_Mid>)  "<OBJ_Angle_Mid>"
  Bus Selector/15 -> Subsystem2/2(<OBJ_Angle_Mid_STD>)  "<OBJ_Angle_Mid_STD>"
  Subsystem2/1(Out1) -> Bus Creator1/9  "Obj_Anage"
  Bus Selector/16 -> Bus Creator1/10  "<OBJ_Inv_TTC>"
  Bus Selector/17 -> Bus Creator1/11  "<OBJ_Inv_TTC_STD>"
  Bus Selector/18 -> Subsystem3/1(<OBJ_Abs_Long_Acc>)  "<OBJ_Abs_Long_Acc>"
  Bus Selector/19 -> Subsystem3/2(<OBJ_Abs_Long_Acc_STD>)  "<OBJ_Abs_Long_Acc_STD>"
  Bus Selector/20 -> Subsystem3/3(<OBJ_Abs_Lat_Acc>)  "<OBJ_Abs_Lat_Acc>"
  Bus Selector/21 -> Subsystem3/4(<OBJ_Abs_Lat_Acc_STD>)  "<OBJ_Abs_Lat_Acc_STD>"
  Subsystem3/1(Out1) -> Bus Creator1/12  "Obj_Acc"
  Constant/1 -> Bus Creator1/13  "existProb"
  Bus Selector/22 -> Subsystem4/1(<OBJ_Length>)  "<OBJ_Length>"
  Bus Selector/23 -> Subsystem4/2(<OBJ_Width>)  "<OBJ_Width>"
  Bus Selector/24 -> Subsystem4/3(<OBJ_Height>)  "<OBJ_Height>"
  Subsystem4/1(Out1) -> Bus Creator1/14  "Obj_BoxSize"
  Constant1/1 -> Bus Creator1/15  "AngelOfObj"
  Subsystem5/1(reserved1) -> Bus Creator1/16
  Bus Selector/25 -> Bus Creator1/17  "<OBJ_Heading>"
  Constant2/1 -> Bus Creator1/18
  Constant3/1 -> Bus Creator1/19
  Constant4/1 -> Bus Creator1/20
  Subsystem6/1(reserved2) -> Bus Creator1/21
  EyeQ4_Obj_01/1 -> Bus Selector/1
  Bus Creator1/1 -> Obj_01_st/1
  Data Type Conversion/1 -> Bus Creator1/1
  Data Type Conversion3/1 -> Bus Creator1/6  "Obj_TypeConf"
  Bus Selector/2 -> Subsystem7/1(<OBJ_Measuring_Status>)  "<OBJ_Measuring_Status>"
  Subsystem7/1(Obj_Status) -> Bus Creator1/2  "Obj_Status"
  Bus Selector/4 -> Subsystem8/1(<OBJ_Object_Class>)  "<OBJ_Object_Class>"
  Subsystem8/1(Obj_Type) -> Bus Creator1/5  "Obj_Type"

== system fusionAlg/FUSION /FUS_DataAdapter/VisionAdapter/ObjAdapter/Obj_8 ==
  EyeQ4_Obj_01 : Inport
  Bus Creator1 : BusCreator  Inputs=21  OutDataTypeStr=Bus: FUS_VISION_OBJ_ST
      settings: InheritFromInputs=off
  Bus Selector : BusSelector  OutputSignals=OBJ_ID,OBJ_Measuring_Status,OBJ_Object_Age,OBJ_Object_Class,OBJ_Class_Probability,OBJ_Lat_Distance,OBJ_Lat_Distance_STD,OBJ_Long_Distance,OBJ_Long_Distance_STD,OBJ_Abs_Long_Velocity,OBJ_Abs_Long_Velocity_STD,OBJ_Abs_Lat_Velocity,OBJ_Abs_Lat_Velocity_STD,OBJ_Angle_Mid,OBJ_Angle_Mid_STD,OBJ_Inv_TTC,OBJ_Inv_TTC_STD,OBJ_Abs_Long_Acc,OBJ_Abs_Long_Acc_STD,OBJ_Abs_Lat_Acc,OBJ_Abs_Lat_Acc_STD,OBJ_Length,OBJ_Width,OBJ_Height,OBJ_Heading
  Constant : Constant  OutDataTypeStr=single
  Constant1 : Constant  Value=0  OutDataTypeStr=uint8
  Constant2 : Constant  OutDataTypeStr=single
  Constant3 : Constant  Value=0  OutDataTypeStr=single
  Constant4 : Constant  Value=0  OutDataTypeStr=single
  Data Type Conversion : DataTypeConversion  OutDataTypeStr=uint32
  Data Type Conversion3 : DataTypeConversion  OutDataTypeStr=uint32
  Obj_01_Agge : Subsystem
  Obj_01_boundarhy : Subsystem
  Subsystem : Subsystem
  Subsystem1 : Subsystem
  Subsystem2 : Subsystem
  Subsystem3 : Subsystem
  Subsystem4 : Subsystem
  Subsystem5 : Subsystem
  Subsystem6 : Subsystem
  Subsystem7 : Subsystem
  Subsystem8 : Subsystem
  Obj_01_st : Outport  OutDataTypeStr=Bus: FUS_VISION_OBJ_ST
  wires:
  Bus Selector/1 -> Data Type Conversion/1  "<OBJ_ID>"
  Bus Selector/3 -> Obj_01_Agge/1(<OBJ_Object_Age>)  "<OBJ_Object_Age>"
  Obj_01_Agge/1(Obj_01_Age) -> Bus Creator1/3  "Obj_Age"
  Obj_01_boundarhy/1(Obj_01_boundary) -> Bus Creator1/4  "Obj_Boundary"
  Bus Selector/5 -> Data Type Conversion3/1  "<OBJ_Class_Probability>"
  Bus Selector/6 -> Subsystem/1(<OBJ_Lat_Distance>)  "<OBJ_Lat_Distance>"
  Bus Selector/7 -> Subsystem/2(<OBJ_Lat_Distance_STD>)  "<OBJ_Lat_Distance_STD>"
  Bus Selector/8 -> Subsystem/3(<OBJ_Long_Distance>)  "<OBJ_Long_Distance>"
  Bus Selector/9 -> Subsystem/4(<OBJ_Long_Distance_STD>)  "<OBJ_Long_Distance_STD>"
  Subsystem/1(Obj_01_coordinate) -> Bus Creator1/7  "Obj_Coor"
  Bus Selector/10 -> Subsystem1/1(<OBJ_Abs_Long_Velocity>)  "<OBJ_Abs_Long_Velocity>"
  Bus Selector/11 -> Subsystem1/2(<OBJ_Abs_Long_Velocity_STD>)  "<OBJ_Abs_Long_Velocity_STD>"
  Bus Selector/12 -> Subsystem1/3(<OBJ_Abs_Lat_Velocity>)  "<OBJ_Abs_Lat_Velocity>"
  Bus Selector/13 -> Subsystem1/4(<OBJ_Abs_Lat_Velocity_STD>)  "<OBJ_Abs_Lat_Velocity_STD>"
  Subsystem1/1(Out1) -> Bus Creator1/8  "Obj_Vel"
  Bus Selector/14 -> Subsystem2/1(<OBJ_Angle_Mid>)  "<OBJ_Angle_Mid>"
  Bus Selector/15 -> Subsystem2/2(<OBJ_Angle_Mid_STD>)  "<OBJ_Angle_Mid_STD>"
  Subsystem2/1(Out1) -> Bus Creator1/9  "Obj_Anage"
  Bus Selector/16 -> Bus Creator1/10  "<OBJ_Inv_TTC>"
  Bus Selector/17 -> Bus Creator1/11  "<OBJ_Inv_TTC_STD>"
  Bus Selector/18 -> Subsystem3/1(<OBJ_Abs_Long_Acc>)  "<OBJ_Abs_Long_Acc>"
  Bus Selector/19 -> Subsystem3/2(<OBJ_Abs_Long_Acc_STD>)  "<OBJ_Abs_Long_Acc_STD>"
  Bus Selector/20 -> Subsystem3/3(<OBJ_Abs_Lat_Acc>)  "<OBJ_Abs_Lat_Acc>"
  Bus Selector/21 -> Subsystem3/4(<OBJ_Abs_Lat_Acc_STD>)  "<OBJ_Abs_Lat_Acc_STD>"
  Subsystem3/1(Out1) -> Bus Creator1/12  "Obj_Acc"
  Constant/1 -> Bus Creator1/13  "existProb"
  Bus Selector/22 -> Subsystem4/1(<OBJ_Length>)  "<OBJ_Length>"
  Bus Selector/23 -> Subsystem4/2(<OBJ_Width>)  "<OBJ_Width>"
  Bus Selector/24 -> Subsystem4/3(<OBJ_Height>)  "<OBJ_Height>"
  Subsystem4/1(Out1) -> Bus Creator1/14  "Obj_BoxSize"
  Constant1/1 -> Bus Creator1/15  "AngelOfObj"
  Subsystem5/1(reserved1) -> Bus Creator1/16
  Bus Selector/25 -> Bus Creator1/17  "<OBJ_Heading>"
  Constant2/1 -> Bus Creator1/18
  Constant3/1 -> Bus Creator1/19
  Constant4/1 -> Bus Creator1/20
  Subsystem6/1(reserved2) -> Bus Creator1/21
  EyeQ4_Obj_01/1 -> Bus Selector/1
  Bus Creator1/1 -> Obj_01_st/1
  Data Type Conversion/1 -> Bus Creator1/1
  Data Type Conversion3/1 -> Bus Creator1/6  "Obj_TypeConf"
  Bus Selector/2 -> Subsystem7/1(<OBJ_Measuring_Status>)  "<OBJ_Measuring_Status>"
  Subsystem7/1(Obj_Status) -> Bus Creator1/2  "Obj_Status"
  Bus Selector/4 -> Subsystem8/1(<OBJ_Object_Class>)  "<OBJ_Object_Class>"
  Subsystem8/1(Obj_Type) -> Bus Creator1/5  "Obj_Type"

== system fusionAlg/FUSION /FUS_DataAdapter/VisionAdapter/ObjAdapter/Obj_9 ==
  EyeQ4_Obj_01 : Inport
  Bus Creator1 : BusCreator  Inputs=21  OutDataTypeStr=Bus: FUS_VISION_OBJ_ST
      settings: InheritFromInputs=off
  Bus Selector : BusSelector  OutputSignals=OBJ_ID,OBJ_Measuring_Status,OBJ_Object_Age,OBJ_Object_Class,OBJ_Class_Probability,OBJ_Lat_Distance,OBJ_Lat_Distance_STD,OBJ_Long_Distance,OBJ_Long_Distance_STD,OBJ_Abs_Long_Velocity,OBJ_Abs_Long_Velocity_STD,OBJ_Abs_Lat_Velocity,OBJ_Abs_Lat_Velocity_STD,OBJ_Angle_Mid,OBJ_Angle_Mid_STD,OBJ_Inv_TTC,OBJ_Inv_TTC_STD,OBJ_Abs_Long_Acc,OBJ_Abs_Long_Acc_STD,OBJ_Abs_Lat_Acc,OBJ_Abs_Lat_Acc_STD,OBJ_Length,OBJ_Width,OBJ_Height,OBJ_Heading
  Constant : Constant  OutDataTypeStr=single
  Constant1 : Constant  Value=0  OutDataTypeStr=uint8
  Constant2 : Constant  OutDataTypeStr=single
  Constant3 : Constant  Value=0  OutDataTypeStr=single
  Constant4 : Constant  Value=0  OutDataTypeStr=single
  Data Type Conversion : DataTypeConversion  OutDataTypeStr=uint32
  Data Type Conversion3 : DataTypeConversion  OutDataTypeStr=uint32
  Obj_01_Agge : Subsystem
  Obj_01_boundarhy : Subsystem
  Subsystem : Subsystem
  Subsystem1 : Subsystem
  Subsystem2 : Subsystem
  Subsystem3 : Subsystem
  Subsystem4 : Subsystem
  Subsystem5 : Subsystem
  Subsystem6 : Subsystem
  Subsystem7 : Subsystem
  Subsystem8 : Subsystem
  Obj_01_st : Outport  OutDataTypeStr=Bus: FUS_VISION_OBJ_ST
  wires:
  Bus Selector/1 -> Data Type Conversion/1  "<OBJ_ID>"
  Bus Selector/3 -> Obj_01_Agge/1(<OBJ_Object_Age>)  "<OBJ_Object_Age>"
  Obj_01_Agge/1(Obj_01_Age) -> Bus Creator1/3  "Obj_Age"
  Obj_01_boundarhy/1(Obj_01_boundary) -> Bus Creator1/4  "Obj_Boundary"
  Bus Selector/5 -> Data Type Conversion3/1  "<OBJ_Class_Probability>"
  Bus Selector/6 -> Subsystem/1(<OBJ_Lat_Distance>)  "<OBJ_Lat_Distance>"
  Bus Selector/7 -> Subsystem/2(<OBJ_Lat_Distance_STD>)  "<OBJ_Lat_Distance_STD>"
  Bus Selector/8 -> Subsystem/3(<OBJ_Long_Distance>)  "<OBJ_Long_Distance>"
  Bus Selector/9 -> Subsystem/4(<OBJ_Long_Distance_STD>)  "<OBJ_Long_Distance_STD>"
  Subsystem/1(Obj_01_coordinate) -> Bus Creator1/7  "Obj_Coor"
  Bus Selector/10 -> Subsystem1/1(<OBJ_Abs_Long_Velocity>)  "<OBJ_Abs_Long_Velocity>"
  Bus Selector/11 -> Subsystem1/2(<OBJ_Abs_Long_Velocity_STD>)  "<OBJ_Abs_Long_Velocity_STD>"
  Bus Selector/12 -> Subsystem1/3(<OBJ_Abs_Lat_Velocity>)  "<OBJ_Abs_Lat_Velocity>"
  Bus Selector/13 -> Subsystem1/4(<OBJ_Abs_Lat_Velocity_STD>)  "<OBJ_Abs_Lat_Velocity_STD>"
  Subsystem1/1(Out1) -> Bus Creator1/8  "Obj_Vel"
  Bus Selector/14 -> Subsystem2/1(<OBJ_Angle_Mid>)  "<OBJ_Angle_Mid>"
  Bus Selector/15 -> Subsystem2/2(<OBJ_Angle_Mid_STD>)  "<OBJ_Angle_Mid_STD>"
  Subsystem2/1(Out1) -> Bus Creator1/9  "Obj_Anage"
  Bus Selector/16 -> Bus Creator1/10  "<OBJ_Inv_TTC>"
  Bus Selector/17 -> Bus Creator1/11  "<OBJ_Inv_TTC_STD>"
  Bus Selector/18 -> Subsystem3/1(<OBJ_Abs_Long_Acc>)  "<OBJ_Abs_Long_Acc>"
  Bus Selector/19 -> Subsystem3/2(<OBJ_Abs_Long_Acc_STD>)  "<OBJ_Abs_Long_Acc_STD>"
  Bus Selector/20 -> Subsystem3/3(<OBJ_Abs_Lat_Acc>)  "<OBJ_Abs_Lat_Acc>"
  Bus Selector/21 -> Subsystem3/4(<OBJ_Abs_Lat_Acc_STD>)  "<OBJ_Abs_Lat_Acc_STD>"
  Subsystem3/1(Out1) -> Bus Creator1/12  "Obj_Acc"
  Constant/1 -> Bus Creator1/13  "existProb"
  Bus Selector/22 -> Subsystem4/1(<OBJ_Length>)  "<OBJ_Length>"
  Bus Selector/23 -> Subsystem4/2(<OBJ_Width>)  "<OBJ_Width>"
  Bus Selector/24 -> Subsystem4/3(<OBJ_Height>)  "<OBJ_Height>"
  Subsystem4/1(Out1) -> Bus Creator1/14  "Obj_BoxSize"
  Constant1/1 -> Bus Creator1/15  "AngelOfObj"
  Subsystem5/1(reserved1) -> Bus Creator1/16
  Bus Selector/25 -> Bus Creator1/17  "<OBJ_Heading>"
  Constant2/1 -> Bus Creator1/18
  Constant3/1 -> Bus Creator1/19
  Constant4/1 -> Bus Creator1/20
  Subsystem6/1(reserved2) -> Bus Creator1/21
  EyeQ4_Obj_01/1 -> Bus Selector/1
  Bus Creator1/1 -> Obj_01_st/1
  Data Type Conversion/1 -> Bus Creator1/1
  Data Type Conversion3/1 -> Bus Creator1/6  "Obj_TypeConf"
  Bus Selector/2 -> Subsystem7/1(<OBJ_Measuring_Status>)  "<OBJ_Measuring_Status>"
  Subsystem7/1(Obj_Status) -> Bus Creator1/2  "Obj_Status"
  Bus Selector/4 -> Subsystem8/1(<OBJ_Object_Class>)  "<OBJ_Object_Class>"
  Subsystem8/1(Obj_Type) -> Bus Creator1/5  "Obj_Type"

== system fusionAlg/FUSION /FUS_DataAdapter/VisionAdapter/ObjAdapter/Obj_reserved1 ==
  Bus Creator : BusCreator  Inputs=3  OutDataTypeStr=Bus: FUS_VISOBJ_UINT8_RESERVED_ST
      settings: InheritFromInputs=off
  Constant1 : Constant  Value=0  OutDataTypeStr=uint8
  Constant2 : Constant  Value=0  OutDataTypeStr=uint8
  Constant3 : Constant  Value=0  OutDataTypeStr=uint8
  reserved1 : Outport
  wires:
  Bus Creator/1 -> reserved1/1
  Constant2/1 -> Bus Creator/1
  Constant1/1 -> Bus Creator/2
  Constant3/1 -> Bus Creator/3

== system fusionAlg/FUSION /FUS_DataAdapter/VisionAdapter/ObjAdapter/Subsystem6 ==
  Bus Creator : BusCreator  Inputs=2  OutDataTypeStr=Bus: FUS_VISOBJ_UINT32_RESERVED_ST
      settings: InheritFromInputs=off
  Constant5 : Constant  Value=0  OutDataTypeStr=uint32
  Constant6 : Constant  Value=0  OutDataTypeStr=uint32
  reserved2 : Outport
  wires:
  Constant5/1 -> Bus Creator/1
  Bus Creator/1 -> reserved2/1
  Constant6/1 -> Bus Creator/2

== system fusionAlg/FUSION /FUS_DataAdapter/VisionAdapter/RoadEdgeAdapter/RoadEdgeProtAAdapter ==
  <RoadEdgeProtA> : Inport
  Bus Creator1 : BusCreator  Inputs=14  OutDataTypeStr=Bus: FUS_EYEQ4_ROADEDGE_PROT_ST  NonVirtualBus=on
      settings: InheritFromInputs=off
  Bus Selector : BusSelector  OutputSignals=LRE_Age,LRE_ExistProb,LRE_Type,LRE_ID,LRE_LineC0,LRE_LineC1,LRE_LineC2,LRE_LineC3,LRE_Start,LRE_End,LRE_Side,LRE_Height,LRE_Height_STD,LRE_Index
  Data Type Conversion{,1..4} (5 alike) : DataTypeConversion  OutDataTypeStr=uint32
  RoadEdgeProtA : Outport
  wires:
  <RoadEdgeProtA>/1 -> Bus Selector/1
  Bus Creator1/1 -> RoadEdgeProtA/1
  Bus Selector/1 -> Data Type Conversion/1  "<LRE_Age>"
  Bus Selector/2 -> Bus Creator1/2  "<LRE_ExistProb>"
  Bus Selector/3 -> Data Type Conversion1/1  "<LRE_Type>"
  Bus Selector/4 -> Data Type Conversion2/1  "<LRE_ID>"
  Bus Selector/5 -> Bus Creator1/5  "<LRE_LineC0>"
  Bus Selector/6 -> Bus Creator1/6  "<LRE_LineC1>"
  Bus Selector/7 -> Bus Creator1/7  "<LRE_LineC2>"
  Bus Selector/8 -> Bus Creator1/8  "<LRE_LineC3>"
  Bus Selector/9 -> Bus Creator1/9  "<LRE_Start>"
  Bus Selector/10 -> Bus Creator1/10  "<LRE_End>"
  Bus Selector/11 -> Data Type Conversion3/1  "<LRE_Side>"
  Bus Selector/12 -> Bus Creator1/12  "<LRE_Height>"
  Bus Selector/13 -> Bus Creator1/13  "<LRE_Height_STD>"
  Bus Selector/14 -> Data Type Conversion4/1  "<LRE_Index>"
  Data Type Conversion/1 -> Bus Creator1/1  "age"
  Data Type Conversion1/1 -> Bus Creator1/3  "type"
  Data Type Conversion2/1 -> Bus Creator1/4  "id"
  Data Type Conversion3/1 -> Bus Creator1/11  "side"
  Data Type Conversion4/1 -> Bus Creator1/14  "index"

== system fusionAlg/FUSION /FUS_DataAdapter/VisionAdapter/RoadEdgeAdapter/RoadEdgeProtBAdapter ==
  <RoadEdgeProtB> : Inport
  Bus Creator1 : BusCreator  Inputs=14  OutDataTypeStr=Bus: FUS_EYEQ4_ROADEDGE_PROT_ST  NonVirtualBus=on
      settings: InheritFromInputs=off
  Bus Selector : BusSelector  OutputSignals=LRE_Age,LRE_ExistProb,LRE_Type,LRE_ID,LRE_LineC0,LRE_LineC1,LRE_LineC2,LRE_LineC3,LRE_Start,LRE_End,LRE_Side,LRE_Height,LRE_Height_STD,LRE_Index
  Data Type Conversion{,1..4} (5 alike) : DataTypeConversion  OutDataTypeStr=uint32
  RoadEdgeProtB : Outport
  wires:
  <RoadEdgeProtB>/1 -> Bus Selector/1
  Bus Creator1/1 -> RoadEdgeProtB/1
  Bus Selector/1 -> Data Type Conversion/1  "<LRE_Age>"
  Bus Selector/2 -> Bus Creator1/2  "<LRE_ExistProb>"
  Bus Selector/3 -> Data Type Conversion1/1  "<LRE_Type>"
  Bus Selector/4 -> Data Type Conversion2/1  "<LRE_ID>"
  Bus Selector/5 -> Bus Creator1/5  "<LRE_LineC0>"
  Bus Selector/6 -> Bus Creator1/6  "<LRE_LineC1>"
  Bus Selector/7 -> Bus Creator1/7  "<LRE_LineC2>"
  Bus Selector/8 -> Bus Creator1/8  "<LRE_LineC3>"
  Bus Selector/9 -> Bus Creator1/9  "<LRE_Start>"
  Bus Selector/10 -> Bus Creator1/10  "<LRE_End>"
  Bus Selector/11 -> Data Type Conversion3/1  "<LRE_Side>"
  Bus Selector/12 -> Bus Creator1/12  "<LRE_Height>"
  Bus Selector/13 -> Bus Creator1/13  "<LRE_Height_STD>"
  Bus Selector/14 -> Data Type Conversion4/1  "<LRE_Index>"
  Data Type Conversion/1 -> Bus Creator1/1  "age"
  Data Type Conversion1/1 -> Bus Creator1/3  "type"
  Data Type Conversion2/1 -> Bus Creator1/4  "id"
  Data Type Conversion3/1 -> Bus Creator1/11  "side"
  Data Type Conversion4/1 -> Bus Creator1/14  "index"

== system fusionAlg/FUSION /FUS_DataAdapter/VisionAdapter/RoadEdgeAdapter/RoadEdgeProtCAdapter ==
  <RoadEdgeProtC> : Inport
  Bus Creator1 : BusCreator  Inputs=14  OutDataTypeStr=Bus: FUS_EYEQ4_ROADEDGE_PROT_ST  NonVirtualBus=on
      settings: InheritFromInputs=off
  Bus Selector : BusSelector  OutputSignals=LRE_Age,LRE_ExistProb,LRE_Type,LRE_ID,LRE_LineC0,LRE_LineC1,LRE_LineC2,LRE_LineC3,LRE_Start,LRE_End,LRE_Side,LRE_Height,LRE_Height_STD,LRE_Index
  Data Type Conversion{,1..4} (5 alike) : DataTypeConversion  OutDataTypeStr=uint32
  RoadEdgeProtC : Outport
  wires:
  <RoadEdgeProtC>/1 -> Bus Selector/1
  Bus Creator1/1 -> RoadEdgeProtC/1
  Bus Selector/1 -> Data Type Conversion/1  "<LRE_Age>"
  Bus Selector/2 -> Bus Creator1/2  "<LRE_ExistProb>"
  Bus Selector/3 -> Data Type Conversion1/1  "<LRE_Type>"
  Bus Selector/4 -> Data Type Conversion2/1  "<LRE_ID>"
  Bus Selector/5 -> Bus Creator1/5  "<LRE_LineC0>"
  Bus Selector/6 -> Bus Creator1/6  "<LRE_LineC1>"
  Bus Selector/7 -> Bus Creator1/7  "<LRE_LineC2>"
  Bus Selector/8 -> Bus Creator1/8  "<LRE_LineC3>"
  Bus Selector/9 -> Bus Creator1/9  "<LRE_Start>"
  Bus Selector/10 -> Bus Creator1/10  "<LRE_End>"
  Bus Selector/11 -> Data Type Conversion3/1  "<LRE_Side>"
  Bus Selector/12 -> Bus Creator1/12  "<LRE_Height>"
  Bus Selector/13 -> Bus Creator1/13  "<LRE_Height_STD>"
  Bus Selector/14 -> Data Type Conversion4/1  "<LRE_Index>"
  Data Type Conversion/1 -> Bus Creator1/1  "age"
  Data Type Conversion1/1 -> Bus Creator1/3  "type"
  Data Type Conversion2/1 -> Bus Creator1/4  "id"
  Data Type Conversion3/1 -> Bus Creator1/11  "side"
  Data Type Conversion4/1 -> Bus Creator1/14  "index"

== system fusionAlg/FUSION /FUS_DataAdapter/VisionAdapter/RoadEdgeAdapter/RoadEdgeProtHeaderAdapter ==
  <RoadEdgeProtHeader> : Inport
  Bus Creator1 : BusCreator  Inputs=14  OutDataTypeStr=Bus: FUS_EYEQ4_ROADEDGE_PROT_ST  NonVirtualBus=on
      settings: InheritFromInputs=off
  Bus Selector : BusSelector  OutputSignals=LRE_Age,LRE_ExistProb,LRE_Type,LRE_ID,LRE_LineC0,LRE_LineC1,LRE_LineC2,LRE_LineC3,LRE_Start,LRE_End,LRE_Side,LRE_Height,LRE_Height_STD,LRE_Index
  Data Type Conversion{,1..4} (5 alike) : DataTypeConversion  OutDataTypeStr=uint32
  RoadEdgeProtHeader : Outport
  wires:
  <RoadEdgeProtHeader>/1 -> Bus Selector/1
  Bus Creator1/1 -> RoadEdgeProtHeader/1
  Bus Selector/1 -> Data Type Conversion/1  "<LRE_Age>"
  Bus Selector/2 -> Bus Creator1/2  "<LRE_ExistProb>"
  Bus Selector/3 -> Data Type Conversion1/1  "<LRE_Type>"
  Bus Selector/4 -> Data Type Conversion2/1  "<LRE_ID>"
  Bus Selector/5 -> Bus Creator1/5  "<LRE_LineC0>"
  Bus Selector/6 -> Bus Creator1/6  "<LRE_LineC1>"
  Bus Selector/7 -> Bus Creator1/7  "<LRE_LineC2>"
  Bus Selector/8 -> Bus Creator1/8  "<LRE_LineC3>"
  Bus Selector/9 -> Bus Creator1/9  "<LRE_Start>"
  Bus Selector/10 -> Bus Creator1/10  "<LRE_End>"
  Bus Selector/11 -> Data Type Conversion3/1  "<LRE_Side>"
  Bus Selector/12 -> Bus Creator1/12  "<LRE_Height>"
  Bus Selector/13 -> Bus Creator1/13  "<LRE_Height_STD>"
  Bus Selector/14 -> Data Type Conversion4/1  "<LRE_Index>"
  Data Type Conversion/1 -> Bus Creator1/1  "age"
  Data Type Conversion1/1 -> Bus Creator1/3  "type"
  Data Type Conversion2/1 -> Bus Creator1/4  "id"
  Data Type Conversion3/1 -> Bus Creator1/11  "side"
  Data Type Conversion4/1 -> Bus Creator1/14  "index"

== system fusionAlg/FUSION /FusionAlg/BusToBusArray/BusToBusArray/FUS_Obj_1 ==
  <fus_output_01_obj> : Inport
  Bus Creator : BusCreator  Inputs=15  OutDataTypeStr=Bus: FUS_OBJ_TRACK_EST_ST  NonVirtualBus=on
      settings: InheritFromInputs=off
  Bus Creator1 : BusCreator  Inputs=15  OutDataTypeStr=Bus: FUS_OBJ_TRACK_PROP_ST  NonVirtualBus=on
      settings: InheritFromInputs=off
  Bus Creator2 : BusCreator  Inputs=10  OutDataTypeStr=Bus: FUS_OBJ_TRACK_INFO_ST  NonVirtualBus=on
      settings: InheritFromInputs=off
  Bus Creator3 : BusCreator  Inputs=3  OutDataTypeStr=Bus: FUS_OBJ_DATA_ST  NonVirtualBus=on
      settings: InheritFromInputs=off
  Bus Selector : BusSelector  OutputSignals=obj_estimate,obj_property,obj_information
  Bus Selector1 : BusSelector  OutputSignals=longPosition,latPosition,headingAngle,speed,yawRate,longRelativeVelocity,latRelativeVelocity,longAbsoluteVelocity,latAbsoluteVelocity,acceleration,longRelativeAcceleration,latRelativeAcceleration,longAbsoluteAcceleration,latAbsoluteAcceleration,curvature
  Bus Selector2 : BusSelector  OutputSignals=id,fusionSource,motionModel,trackStatus,positionConfidence,fcwConfidence,tjaConfidence,leftNearLaneMarkingConfidence,rightNearLaneMarkingConfidence,visionId,accelerationStdDev,headingAngleStdDev,latPositionStdDev,longPositionStdDev,speedStdDev
  Bus Selector3 : BusSelector  OutputSignals=valid,type,nearestSide,motionPatternCurrent,motionPatternHistory,width,height,length,distanceToleftNearLaneMarking,distanceToRightNearLaneMarking
  BUS_fus_output_01_obj : Outport
  wires:
  <fus_output_01_obj>/1 -> Bus Selector/1
  Bus Selector/1 -> Bus Selector1/1  "<obj_estimate>"
  Bus Selector1/1 -> Bus Creator/1  "<longPosition>"
  Bus Selector1/2 -> Bus Creator/2  "<latPosition>"
  Bus Selector1/4 -> Bus Creator/4  "<speed>"
  Bus Selector1/5 -> Bus Creator/5  "<yawRate>"
  Bus Selector1/6 -> Bus Creator/6  "<longRelativeVelocity>"
  Bus Selector1/3 -> Bus Creator/3  "<headingAngle>"
  Bus Selector1/7 -> Bus Creator/7  "<latRelativeVelocity>"
  Bus Selector/2 -> Bus Selector2/1  "<obj_property>"
  Bus Selector/3 -> Bus Selector3/1  "<obj_information>"
  Bus Selector2/1 -> Bus Creator1/1  "<id>"
  Bus Selector2/2 -> Bus Creator1/2  "<fusionSource>"
  Bus Selector2/3 -> Bus Creator1/3  "<motionModel>"
  Bus Selector2/4 -> Bus Creator1/4  "<trackStatus>"
  Bus Selector2/6 -> Bus Creator1/6  "<fcwConfidence>"
  Bus Selector2/11 -> Bus Creator1/11  "<accelerationStdDev>"
  Bus Selector2/12 -> Bus Creator1/12  "<headingAngleStdDev>"
  Bus Selector2/13 -> Bus Creator1/13  "<latPositionStdDev>"
  Bus Selector2/14 -> Bus Creator1/14  "<longPositionStdDev>"
  Bus Selector2/15 -> Bus Creator1/15  "<speedStdDev>"
  Bus Selector2/9 -> Bus Creator1/9  "<rightNearLaneMarkingConfidence>"
  Bus Selector2/8 -> Bus Creator1/8  "<leftNearLaneMarkingConfidence>"
  Bus Selector2/10 -> Bus Creator1/10  "<visionId>"
  Bus Selector2/5 -> Bus Creator1/5  "<positionConfidence>"
  Bus Selector2/7 -> Bus Creator1/7  "<tjaConfidence>"
  Bus Selector3/1 -> Bus Creator2/1  "<valid>"
  Bus Selector3/2 -> Bus Creator2/2  "<type>"
  Bus Selector3/3 -> Bus Creator2/3  "<nearestSide>"
  Bus Selector3/4 -> Bus Creator2/4  "<motionPatternCurrent>"
  Bus Selector3/5 -> Bus Creator2/5  "<motionPatternHistory>"
  Bus Selector3/6 -> Bus Creator2/6  "<width>"
  Bus Selector3/7 -> Bus Creator2/7  "<height>"
  Bus Selector3/8 -> Bus Creator2/8  "<length>"
  Bus Selector3/9 -> Bus Creator2/9  "<distanceToleftNearLaneMarking>"
  Bus Creator/1 -> Bus Creator3/1
  Bus Creator1/1 -> Bus Creator3/2
  Bus Creator2/1 -> Bus Creator3/3
  Bus Creator3/1 -> BUS_fus_output_01_obj/1
  Bus Selector3/10 -> Bus Creator2/10  "<distanceToRightNearLaneMarking>"
  Bus Selector1/8 -> Bus Creator/8  "<longAbsoluteVelocity>"
  Bus Selector1/9 -> Bus Creator/9  "<latAbsoluteVelocity>"
  Bus Selector1/10 -> Bus Creator/10  "<acceleration>"
  Bus Selector1/11 -> Bus Creator/11  "<longRelativeAcceleration>"
  Bus Selector1/12 -> Bus Creator/12  "<latRelativeAcceleration>"
  Bus Selector1/13 -> Bus Creator/13  "<longAbsoluteAcceleration>"
  Bus Selector1/14 -> Bus Creator/14  "<latAbsoluteAcceleration>"
  Bus Selector1/15 -> Bus Creator/15  "<curvature>"
